simulink model "ihc_lowpass_filter"  (R2020b)
settings: Solver=FixedStepDiscrete  StartTime=0.0  StopTime=stopTime  RelTol=1e-3
InitFcn:
  | initCallback
StopFcn:
  | stopCallback
values from neighbouring files (symbols this model uses):
  IHCLPcoeffs = [  gainihc*c2LPihc gainihc*c2LPihc 0 1 -c1LPihc 0 ... (first row only)    [modelparameters.m]
undefined symbols (not defined in the file or in its folder): mp
settings Model: Creator=Ross  LastModifiedBy=conno
settings DataIOCC: ReturnWorkspaceOutputs=off
settings OptimizationCC: BlockReduction=off  ConditionallyExecuteInputs=off  DefaultParameterBehavior=Inlined
settings DebuggingCC: ReadBeforeWriteMsg=DisableAll  WriteAfterWriteMsg=DisableAll  WriteAfterReadMsg=DisableAll  AlgebraicLoopMsg=error  MultiTaskDSMMsg=none  SingleTaskRateTransMsg=error  PregeneratedLibrarySubsystemCodeDiagnostic=none  ArithmeticOperatorsInVariantConditions=warning
settings HardwareCC: ProdBitPerPointer=32  ProdBitPerSizeT=32  ProdBitPerPtrDiffT=32  ProdLargestAtomicFloat=None  ProdIntDivRoundTo=Undefined  ProdEndianess=Unspecified  ProdWordSize=32  ProdHWDeviceType=ASIC/FPGA->ASIC/FPGA  TargetBitPerPointer=64  TargetBitPerSizeT=64  TargetBitPerPtrDiffT=64  TargetLongLongMode=on  TargetIntDivRoundTo=Zero  TargetEndianess=LittleEndian  TargetWordSize=64  TargetHWDeviceType=Custom Processor->MATLAB Host Computer  ProdEqTarget=off
settings ModelReferenceCC: UpdateModelReferenceTargets=IfOutOfDate
settings SFSimCC: SFSimEcho=off  SimUseLocalCustomCode=off  CustomCodeUndefinedFunction=UseInterfaceOnly
settings RTWCC: RTWUseLocalCustomCode=off

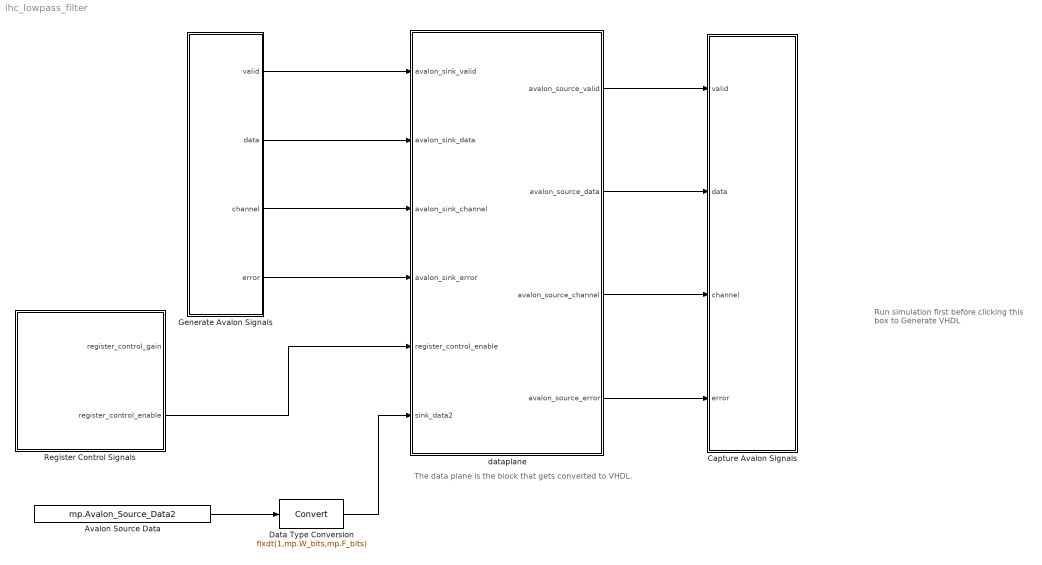
== system ihc_lowpass_filter ==
  note: The data plane is the block that gets converted to VHDL.
  note: Run simulation first
      | before clicking this box to
      | Generate VHDL
  "Avalon Source Data " : FromWorkspace  VariableName=mp.Avalon_Source_Data2  OutDataTypeStr=double  SampleTime=mp.Ts_sim
  Capture Avalon Signals : Subsystem
  Data Type Conversion : DataTypeConversion  OutDataTypeStr=fixdt(1,mp.W_bits,mp.F_bits)
  Generate Avalon Signals : Subsystem
  Register Control Signals : Subsystem
  dataplane : Subsystem  TreatAsAtomicUnit=on
  wires:
  Generate Avalon Signals/2(data) -> dataplane/2(avalon_sink_data)
  Generate Avalon Signals/1(valid) -> dataplane/1(avalon_sink_valid)
  Generate Avalon Signals/3(channel) -> dataplane/3(avalon_sink_channel)
  Generate Avalon Signals/4(error) -> dataplane/4(avalon_sink_error)
  dataplane/2(avalon_source_data) -> Capture Avalon Signals/2(data)
  dataplane/1(avalon_source_valid) -> Capture Avalon Signals/1(valid)
  dataplane/3(avalon_source_channel) -> Capture Avalon Signals/3(channel)
  dataplane/4(avalon_source_error) -> Capture Avalon Signals/4(error)
  Register Control Signals/2(register_control_enable) -> dataplane/5(register_control_enable)
  Data Type Conversion/1 -> dataplane/6(sink_data2)
  "Avalon Source Data "/1 -> Data Type Conversion/1

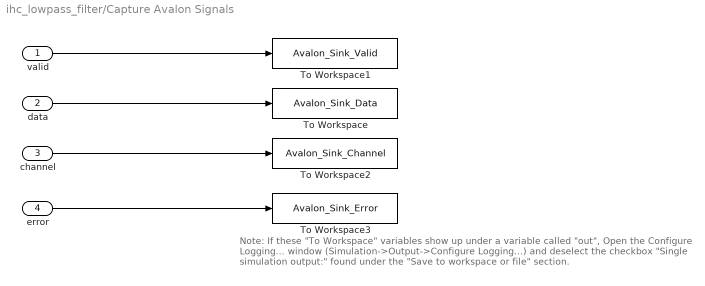
== system ihc_lowpass_filter/Capture Avalon Signals ==
  note: Note:  If these "To Workspace" variables show up under a variable called "out",
      | Open the Configure Logging... window (Simulation->Output->Configure Logging...)
      | and deselect the checkbox "Single simulation output:" found under the "Save to workspace or file" section.
  valid : Inport
  data : Inport  Port=2
  channel : Inport  Port=3
  error : Inport  Port=4
  To Workspace : ToWorkspace  VariableName=Avalon_Sink_Data  SaveFormat=Timeseries  SampleTime=-1
  To Workspace1 : ToWorkspace  VariableName=Avalon_Sink_Valid  SaveFormat=Timeseries  SampleTime=-1
  To Workspace2 : ToWorkspace  VariableName=Avalon_Sink_Channel  SaveFormat=Timeseries  SampleTime=-1
  To Workspace3 : ToWorkspace  VariableName=Avalon_Sink_Error  SaveFormat=Timeseries  SampleTime=-1
  wires:
  data/1 -> To Workspace/1
  valid/1 -> To Workspace1/1
  error/1 -> To Workspace3/1
  channel/1 -> To Workspace2/1

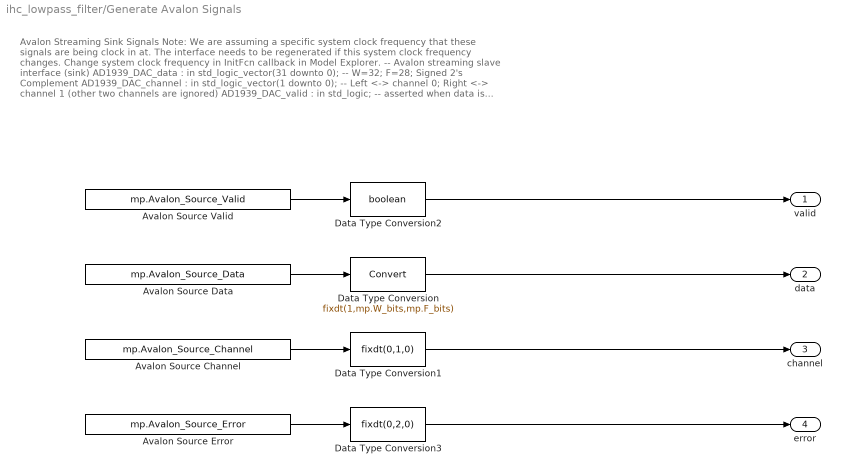
== system ihc_lowpass_filter/Generate Avalon Signals ==
  note: Avalon Streaming Sink Signals
      | Note: We are assuming a specific system clock frequency that these signals are being clock in at.
      | The interface needs to be regenerated if this system clock frequency changes. Change system clock frequency in InitFcn callback in Model Explorer.
      |
      | -- Avalon streaming slave interface (sink)
      | AD1939_DAC_data : in std_logic_vector(31 downto 0); -- W=32; F=28; Signed 2's Complement
      | AD1939_DAC_channel : in std_logic_vector(1 downto 0); -- Left <-> channel 0; Right <-> channel 1 (other two channels are ignored)
      | AD1939_DAC_valid : in std_logic; -- asserted when data is valid
      | AD1939_DAC_error : in std_logic_vector(1 downto 0) -- error channel is ignored, assumed to be error free at this point
      |
      | For more information on the data-channel-valid protocol, s ee chapter 5 in Intel's Avalon Interfaced Specification (p. 40) at https://www.intel.com/content/dam/www/programmable/us/en/pdfs/literature/manual/mnl_avalon_spec.pdf
  Avalon Source Channel : FromWorkspace  VariableName=mp.Avalon_Source_Channel  OutDataTypeStr=double  SampleTime=mp.Ts_sim
  "Avalon Source Data " : FromWorkspace  VariableName=mp.Avalon_Source_Data  OutDataTypeStr=double  SampleTime=mp.Ts_sim
  Avalon Source Error : FromWorkspace  VariableName=mp.Avalon_Source_Error  OutDataTypeStr=double  SampleTime=mp.Ts_sim
  Avalon Source Valid : FromWorkspace  VariableName=mp.Avalon_Source_Valid  OutDataTypeStr=double  SampleTime=mp.Ts_sim
  Data Type Conversion : DataTypeConversion  OutDataTypeStr=fixdt(1,mp.W_bits,mp.F_bits)
  Data Type Conversion1 : DataTypeConversion  OutDataTypeStr=fixdt(0,1,0)
  Data Type Conversion2 : DataTypeConversion  OutDataTypeStr=boolean
  Data Type Conversion3 : DataTypeConversion  OutDataTypeStr=fixdt(0,2,0)
  valid : Outport  VectorParamsAs1DForOutWhenUnconnected=off
  data : Outport  Port=2  VectorParamsAs1DForOutWhenUnconnected=off
  channel : Outport  Port=3  VectorParamsAs1DForOutWhenUnconnected=off
  error : Outport  Port=4  VectorParamsAs1DForOutWhenUnconnected=off
  wires:
  Data Type Conversion1/1 -> channel/1
  Data Type Conversion2/1 -> valid/1
  Avalon Source Error/1 -> Data Type Conversion3/1
  Data Type Conversion/1 -> data/1
  Avalon Source Valid/1 -> Data Type Conversion2/1
  Data Type Conversion3/1 -> error/1
  Avalon Source Channel/1 -> Data Type Conversion1/1
  "Avalon Source Data "/1 -> Data Type Conversion/1

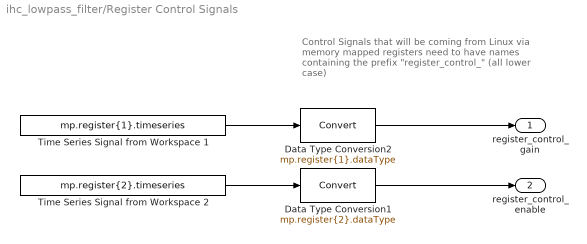
== system ihc_lowpass_filter/Register Control Signals ==
  note: Control Signals that will be coming from Linux via
      | memory mapped registers need to have names
      | containing the prefix "register_control_"
      | (all lower case)
  Data Type Conversion1 : DataTypeConversion  OutDataTypeStr=mp.register{2}.dataType
  Data Type Conversion2 : DataTypeConversion  OutDataTypeStr=mp.register{1}.dataType
  Time Series Signal from Workspace 1 : FromWorkspace  VariableName=mp.register{1}.timeseries  OutDataTypeStr=double  SampleTime=mp.Ts_sim
  Time Series Signal from Workspace 2 : FromWorkspace  VariableName=mp.register{2}.timeseries  OutDataTypeStr=double  SampleTime=mp.Ts_sim
  register_control_gain : Outport  VectorParamsAs1DForOutWhenUnconnected=off
  register_control_enable : Outport  Port=2  VectorParamsAs1DForOutWhenUnconnected=off
  wires:
  Time Series Signal from Workspace 1/1 -> Data Type Conversion2/1
  Data Type Conversion2/1 -> register_control_gain/1
  Data Type Conversion1/1 -> register_control_enable/1
  Time Series Signal from Workspace 2/1 -> Data Type Conversion1/1

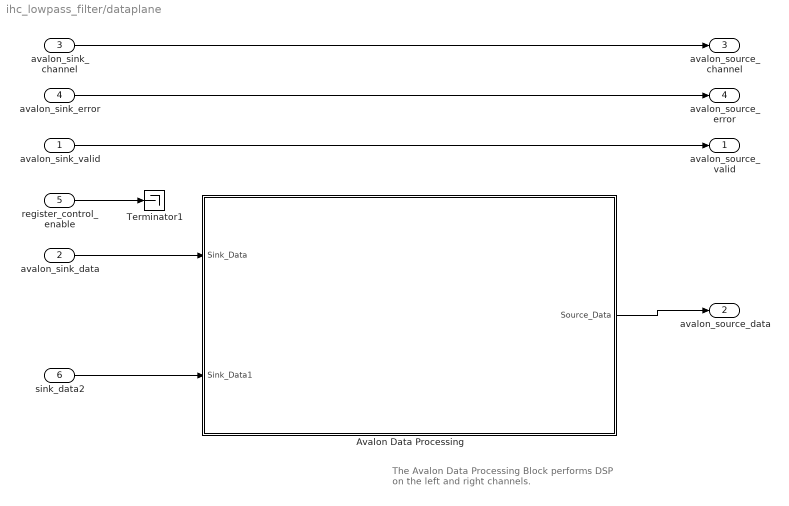
== system ihc_lowpass_filter/dataplane ==
  note: The Avalon Data Processing Block
      | performs DSP on the left and right channels.
  avalon_sink_valid : Inport
  avalon_sink_data : Inport  Port=2
  avalon_sink_channel : Inport  Port=3
  avalon_sink_error : Inport  Port=4
  register_control_enable : Inport  Port=5
  sink_data2 : Inport  Port=6
  Avalon Data Processing : Subsystem  TreatAsAtomicUnit=on
  Terminator1 : Terminator
  avalon_source_valid : Outport  VectorParamsAs1DForOutWhenUnconnected=off
  avalon_source_data : Outport  Port=2  VectorParamsAs1DForOutWhenUnconnected=off
  avalon_source_channel : Outport  Port=3  VectorParamsAs1DForOutWhenUnconnected=off
  avalon_source_error : Outport  Port=4  VectorParamsAs1DForOutWhenUnconnected=off
  wires:
  avalon_sink_error/1 -> avalon_source_error/1
  avalon_sink_valid/1 -> avalon_source_valid/1
  avalon_sink_data/1 -> Avalon Data Processing/1(Sink_Data)
  Avalon Data Processing/1(Source_Data) -> avalon_source_data/1
  avalon_sink_channel/1 -> avalon_source_channel/1
  register_control_enable/1 -> Terminator1/1
  sink_data2/1 -> Avalon Data Processing/2(Sink_Data1)

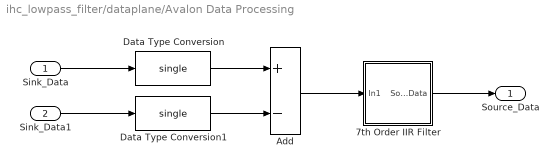
== system ihc_lowpass_filter/dataplane/Avalon Data Processing ==
  Sink_Data : Inport
  Sink_Data1 : Inport  Port=2
  7th Order IIR Filter : Subsystem
  Add : Sum  Inputs=+-  RndMeth=Nearest
  Data Type Conversion : DataTypeConversion  OutDataTypeStr=single
  Data Type Conversion1 : DataTypeConversion  OutDataTypeStr=single
  Source_Data : Outport  InitialOutput=0  VectorParamsAs1DForOutWhenUnconnected=off
  wires:
  Sink_Data/1 -> Data Type Conversion/1
  Data Type Conversion/1 -> Add/1
  Sink_Data1/1 -> Data Type Conversion1/1
  Data Type Conversion1/1 -> Add/2
  Add/1 -> 7th Order IIR Filter/1(In1)
  7th Order IIR Filter/1(Source_Data) -> Source_Data/1

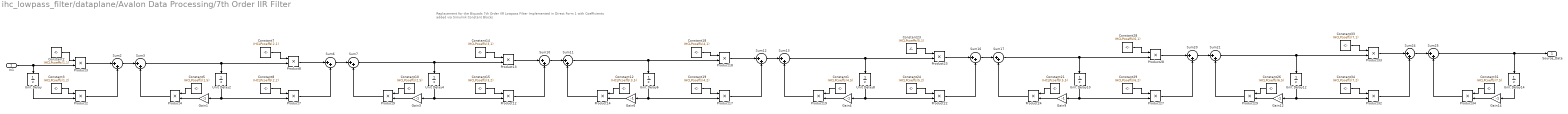
== system ihc_lowpass_filter/dataplane/Avalon Data Processing/7th Order IIR Filter ==
  note: Replacement for the Biquads
      | 7th Order IIR Lowpass Filter Implemented in Direct Form 1 with Coefficients added via Simulink Constant Blocks
  In1 : Inport  OutDataTypeStr=single
  Constant1 : Constant  Value=IHCLPcoeffs(4,5)  OutDataTypeStr=single  SampleTime=-1
  Constant10 : Constant  Value=IHCLPcoeffs(2,5)  OutDataTypeStr=single  SampleTime=-1
  Constant12 : Constant  Value=IHCLPcoeffs(3,5)  OutDataTypeStr=single  SampleTime=-1
  Constant14 : Constant  Value=IHCLPcoeffs(3,1)  OutDataTypeStr=single  SampleTime=-1
  Constant15 : Constant  Value=IHCLPcoeffs(3,2)  OutDataTypeStr=single  SampleTime=-1
  Constant18 : Constant  Value=IHCLPcoeffs(4,1)  OutDataTypeStr=single  SampleTime=-1
  Constant19 : Constant  Value=IHCLPcoeffs(4,2)  OutDataTypeStr=single  SampleTime=-1
  Constant2 : Constant  Value=IHCLPcoeffs(1,1)  OutDataTypeStr=single  SampleTime=-1
  Constant21 : Constant  Value=IHCLPcoeffs(5,5)  OutDataTypeStr=single  SampleTime=-1
  Constant23 : Constant  Value=IHCLPcoeffs(5,1)  OutDataTypeStr=single  SampleTime=-1
  Constant24 : Constant  Value=IHCLPcoeffs(5,2)  OutDataTypeStr=single  SampleTime=-1
  Constant26 : Constant  Value=IHCLPcoeffs(6,5)  OutDataTypeStr=single  SampleTime=-1
  Constant28 : Constant  Value=IHCLPcoeffs(6,1)  OutDataTypeStr=single  SampleTime=-1
  Constant29 : Constant  Value=IHCLPcoeffs(6,2)  OutDataTypeStr=single  SampleTime=-1
  Constant3 : Constant  Value=IHCLPcoeffs(1,2)  OutDataTypeStr=single  SampleTime=-1
  Constant31 : Constant  Value=IHCLPcoeffs(7,5)  OutDataTypeStr=single  SampleTime=-1
  Constant33 : Constant  Value=IHCLPcoeffs(7,1)  OutDataTypeStr=single  SampleTime=-1
  Constant34 : Constant  Value=IHCLPcoeffs(7,2)  OutDataTypeStr=single  SampleTime=-1
  Constant5 : Constant  Value=IHCLPcoeffs(1,5)  OutDataTypeStr=single  SampleTime=-1
  Constant7 : Constant  Value=IHCLPcoeffs(2,1)  OutDataTypeStr=single  SampleTime=-1
  Constant8 : Constant  Value=IHCLPcoeffs(2,2)  OutDataTypeStr=single  SampleTime=-1
  Gain{1,3..4,6,9,12,14} (7 alike) : Gain  Gain=-1
  Product{2..4,7..9,12..14,17..19,22..24,27..29,32..34} (21 alike) : Product
  Sum{2..3,6..7,10..13,16..17,20..21,24..25} (14 alike) : Sum  Inputs=|++
  Unit Delay{,2,4,6,8,10,12,14} (8 alike) : UnitDelay  SampleTime=-1  HasFrameUpgradeWarning=on
  Source_Data : Outport  OutDataTypeStr=single
  wires:
  Constant31/1 -> Product34/1
  Product34/1 -> Sum25/2
  Sum24/1 -> Sum25/1
  Gain14/1 -> Product34/2
  Sum25/1 -> Unit Delay14/1, Source_Data/1
  Product32/1 -> Sum24/2
  Product33/1 -> Sum24/1
  Unit Delay14/1 -> Gain14/1
  Constant34/1 -> Product32/1
  Constant33/1 -> Product33/1
  Constant26/1 -> Product29/1
  Product29/1 -> Sum21/2
  Sum20/1 -> Sum21/1
  Gain12/1 -> Product29/2
  Sum21/1 -> Product33/2, Unit Delay12/1
  Product27/1 -> Sum20/2
  Product28/1 -> Sum20/1
  Unit Delay12/1 -> Gain12/1, Product32/2
  Constant29/1 -> Product27/1
  Constant28/1 -> Product28/1
  Sum12/1 -> Sum13/1
  Constant23/1 -> Product23/1
  Constant2/1 -> Product3/1
  Constant7/1 -> Product8/1
  In1/1 -> Unit Delay/1, Product3/2
  Product8/1 -> Sum6/1
  Constant1/1 -> Product19/1
  Unit Delay4/1 -> Gain3/1, Product12/2
  Product24/1 -> Sum17/2
  Constant24/1 -> Product22/1
  Gain6/1 -> Product14/2
  Sum13/1 -> Product23/2, Unit Delay8/1
  Sum7/1 -> Product13/2, Unit Delay4/1
  Product12/1 -> Sum10/2
  Gain1/1 -> Product4/2
  Product14/1 -> Sum11/2
  Gain4/1 -> Product19/2
  Sum10/1 -> Sum11/1
  Gain9/1 -> Product24/2
  Unit Delay10/1 -> Gain9/1, Product27/2
  Unit Delay6/1 -> Gain6/1, Product17/2
  Product4/1 -> Sum3/2
  Sum11/1 -> Product18/2, Unit Delay6/1
  Product18/1 -> Sum12/1
  Constant15/1 -> Product12/1
  Sum16/1 -> Sum17/1
  Constant19/1 -> Product17/1
  Unit Delay2/1 -> Gain1/1, Product7/2
  Constant21/1 -> Product24/1
  Constant3/1 -> Product2/1
  Product3/1 -> Sum2/1
  Product23/1 -> Sum16/1
  Sum3/1 -> Product8/2, Unit Delay2/1
  Product22/1 -> Sum16/2
  Unit Delay8/1 -> Gain4/1, Product22/2
  Unit Delay/1 -> Product2/2
  Gain3/1 -> Product9/2
  Product17/1 -> Sum12/2
  Product13/1 -> Sum10/1
  Sum17/1 -> Product28/2, Unit Delay10/1
  Constant14/1 -> Product13/1
  Constant12/1 -> Product14/1
  Constant18/1 -> Product18/1
  Product9/1 -> Sum7/2
  Constant5/1 -> Product4/1
  Constant10/1 -> Product9/1
  Product19/1 -> Sum13/2
  Constant8/1 -> Product7/1
  Sum2/1 -> Sum3/1
  Sum6/1 -> Sum7/1
  Product2/1 -> Sum2/2
  Product7/1 -> Sum6/2
